simulink model "ArthCalcStateFlow"  (R2018b)
settings: Solver=FixedStepDiscrete  StartTime=0.0  StopTime=10.0  RelTol=1e-3
settings Model: Creator=dahroug  LastModifiedBy=dahroug
settings OptimizationCC: DefaultParameterBehavior=Inlined  EnhancedBackFolding=on  PassReuseOutputArgsAs=Individual arguments  OptimizeBlockOrder=speed  DifferentSizesBufferReuse=on  OptimizationCustomize=off
settings DebuggingCC: UnderspecifiedInitializationDetection=Classic  MergeDetectMultiDrivingBlocksExec=none  ParameterTunabilityLossMsg=error
settings ModelReferenceCC: PropagateSignalLabelsOutOfModel=off
settings SFSimCC: MATLABDynamicMemAlloc=off
settings RTWCC: SystemTargetFile=ert.tlc  GenCodeOnly=on  TemplateMakefile=ert_default_tmf  GenerateReport=on  IncludeHyperlinkInReport=on  LaunchReport=on  GenerateTraceInfo=on  GenerateTraceReport=on  GenerateTraceReportSl=on  GenerateTraceReportSf=on  GenerateTraceReportEml=on
settings CodeAppCC: ForceParamTrailComments=on  IgnoreCustomStorageClasses=off  OperatorAnnotations=on  SimulinkDataObjDesc=on  SFDataObjDesc=on  InsertBlockDesc=on
settings ERTTargetCC: TargetLangStandard=C99 (ISO)  GenerateSampleERTMain=on  InlinedParameterPlacement=NonHierarchical  ERTCustomFileTemplate=example_file_process.tlc

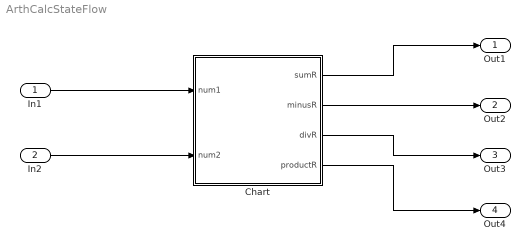
== system ArthCalcStateFlow ==
  In1 : Inport
  In2 : Inport  Port=2
  Chart : Stateflow chart  TreatAsAtomicUnit=on
  Out1 : Outport
  Out2 : Outport  Port=2
  Out3 : Outport  Port=3
  Out4 : Outport  Port=4
  wires:
  In1/1 -> Chart/1(num1)
  In2/1 -> Chart/2(num2)
  Chart/1(sumR) -> Out1/1
  Chart/2(minusR) -> Out2/1
  Chart/3(divR) -> Out3/1
  Chart/4(productR) -> Out4/1

== stateflow chart ArthCalcStateFlow/Chart ==
  state sum [function]
    (default) -> (junction 9) : {sumResult = num1+num2;}
  state minus [function]
    (default) -> (junction 22) : {minusResult = num1-num2;}
  state div [function]
    (default) -> (junction 34)
    (junction 34) -> (junction 44) [order 2] : [num2==0]
    (junction 34) -> (junction 36) [order 1] : {divResult = num1/num2;}
    (junction 44) -> (junction 46) : {divResult=0;}
    (junction 46) -> (junction 36)
    (junction 36) -> (junction 37)
  state product [function]
    (default) -> (junction 43) : {productResult = num1*num2;}
  (default) -> (junction 65) : {
      | sumR = sum(num1,num2);
      | minusR = minus(num1,num2);
      | divR = div(num1,num2);
      | productR =product(num1,num2);
      | }
  data: num1 input uint8; num2 input uint8; sumR output uint8; minusR output uint8; divR output uint8; productR output uint8
